simulink model "Visualisation"  (R2023a)
settings: Solver=VariableStepAuto  StartTime=0.0  StopTime=10.0  RelTol=1e-3
values from neighbouring files (symbols this model uses):
  A_long = inv(P_long) * Q_long    [parameters_ctrl.m]
  B_long = inv(P_long) * R_long    [parameters_ctrl.m]
  C_long = eye(4)    [parameters_ctrl.m]
  D_long = zeros(4,2)    [parameters_ctrl.m]
undefined symbols (not defined in the file or in its folder): A_lat, B_lat, C_lat, D_lat
libraries: simulink x2, vrlib x1
settings Model: Creator=simon  LastModifiedBy=simon
settings OptimizationCC: ReuseModelBlockBuffer=off

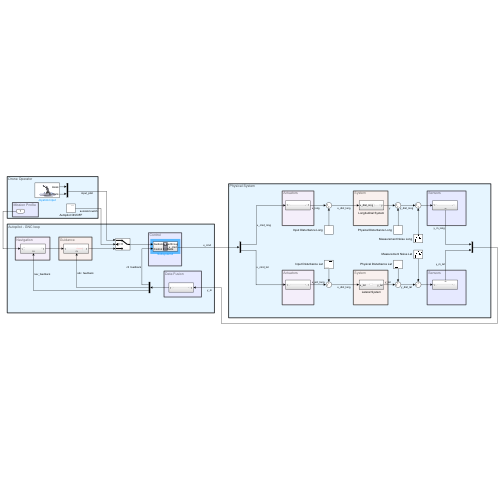
[thumbnail: Simulink's stored preview of the top-level diagram]
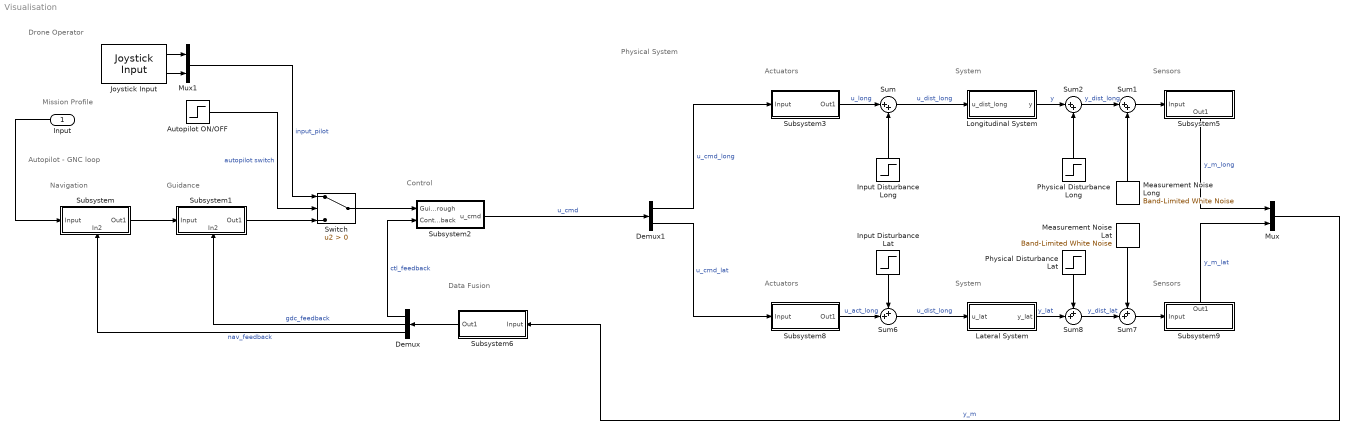
== system Visualisation ==
  note: Drone Operator
  note: Physical System
  note: Autopilot - GNC loop
  note: Navigation
  note: Mission Profile
  note: Guidance
  note: Control
  note: Data Fusion
  note: Actuators
  note: System
  note: Sensors
  note: Sensors
  note: System
  note: Actuators
  Input : Inport
  Autopilot ON/OFF : Step  SampleTime=0
  Demux : Demux  Outputs=3
  Demux1 : Demux  Outputs=2
  Input Disturbance Lat : Step  SampleTime=0
  Input Disturbance Long : Step  SampleTime=0
  Joystick Input : vrlib/Joystick Input  joyid=1  adjustports=on  forcefeed=off
  Lateral System : Subsystem
  Longitudinal System : Subsystem
  Measurement Noise Lat : simulink/Sources/Band-Limited White Noise  Cov=[0.1]  Ts=0.1  seed=[23341]
  Measurement Noise Long : simulink/Sources/Band-Limited White Noise  Cov=[0.1]  Ts=0.1  seed=[23341]
  Mux : Mux  Inputs=2
  Mux1 : Mux  Inputs=2
  Physical Disturbance Lat : Step  SampleTime=0
  Physical Disturbance Long : Step  SampleTime=0
  Subsystem : Subsystem
      settings: PortSchema="{\"entries\":[{\"content\":{\"sides\":[{\"content\":{\"connectorIds\":[\"In1\"]},\"type\":\"ConnectorPlacement.EquallySpacedRectSide\",\"uuid\":\"b55c321e-6281-45a5-aa96-a8b4b9a904a2\"},{\"content\":{\"connectorIds\":[\"Out1\"],\"side\":\"RIGHT\"},\"type\":\"ConnectorPlacement.EquallySpacedRectSide\",\"uuid\":\"1acfb3ee-82d1-4624-97ca-4ff12c3c13a9\"},{\"content\":{\"side\":\"TOP\"},\"type\":\"ConnectorPlacement.EquallySpacedRectSide\",\"uuid\":\"e43a3246-7b87-4c39-ab7c-07bd34ecd1c3\"},{\"content\":{\"connectorIds\":[\"In2\"],\"side\":\"BOTTOM\"},\"type\":\"ConnectorPlacement.EquallySpacedRectSide\",\"uuid\":\"a296ef05-0bf2-440a-9974-10a45cf72fb1\"}]},\"type\":\"ConnectorPlacement.EquallySpacedConnector\",\"uuid\":\"140a1a7e-2a00-4d9b-85bf-b1c0a6988ae3\"}],\"packageUris\":[\"http://schema.mathworks.com/mf0/Connector/R2020b\"],\"version\":\"1.0\"}"
  Subsystem1 : Subsystem
      settings: PortSchema="{\"entries\":[{\"content\":{\"sides\":[{\"content\":{\"connectorIds\":[\"In1\"]},\"type\":\"ConnectorPlacement.EquallySpacedRectSide\",\"uuid\":\"2eb23210-3dea-4b77-a9d4-7110bad0c58c\"},{\"content\":{\"connectorIds\":[\"Out1\"],\"side\":\"RIGHT\"},\"type\":\"ConnectorPlacement.EquallySpacedRectSide\",\"uuid\":\"94c709a1-e7e1-4346-819b-fd02519f91fd\"},{\"content\":{\"connectorIds\":[],\"side\":\"TOP\"},\"type\":\"ConnectorPlacement.EquallySpacedRectSide\",\"uuid\":\"53af2cc2-9550-447d-847d-ecbf9bed457e\"},{\"content\":{\"connectorIds\":[\"In2\"],\"side\":\"BOTTOM\"},\"type\":\"ConnectorPlacement.EquallySpacedRectSide\",\"uuid\":\"c0cb6d07-421f-4c5f-9ed6-902a152412e2\"}]},\"type\":\"ConnectorPlacement.EquallySpacedConnector\",\"uuid\":\"16662f53-7def-47cf-8bdf-f2fc9af7dce9\"}],\"packageUris\":[\"http://schema.mathworks.com/mf0/Connector/R2020b\"],\"version\":\"1.0\"}"
  Subsystem2 : Subsystem
  Subsystem3 : Subsystem
  Subsystem5 : Subsystem
      settings: PortSchema="{\"entries\":[{\"content\":{\"sides\":[{\"content\":{\"connectorIds\":[\"In1\"]},\"type\":\"ConnectorPlacement.EquallySpacedRectSide\",\"uuid\":\"2eb23210-3dea-4b77-a9d4-7110bad0c58c\"},{\"content\":{\"connectorIds\":[],\"side\":\"RIGHT\"},\"type\":\"ConnectorPlacement.EquallySpacedRectSide\",\"uuid\":\"94c709a1-e7e1-4346-819b-fd02519f91fd\"},{\"content\":{\"connectorIds\":[],\"side\":\"TOP\"},\"type\":\"ConnectorPlacement.EquallySpacedRectSide\",\"uuid\":\"53af2cc2-9550-447d-847d-ecbf9bed457e\"},{\"content\":{\"connectorIds\":[\"Out1\"],\"side\":\"BOTTOM\"},\"type\":\"ConnectorPlacement.EquallySpacedRectSide\",\"uuid\":\"b1df5d71-6836-4899-8e9d-10bba38a631d\"}]},\"type\":\"ConnectorPlacement.EquallySpacedConnector\",\"uuid\":\"16662f53-7def-47cf-8bdf-f2fc9af7dce9\"}],\"packageUris\":[\"http://schema.mathworks.com/mf0/Connector/R2020b\"],\"version\":\"1.0\"}"
  Subsystem6 : Subsystem
  Subsystem8 : Subsystem
  Subsystem9 : Subsystem
      settings: PortSchema="{\"entries\":[{\"content\":{\"sides\":[{\"content\":{\"connectorIds\":[\"In1\"]},\"type\":\"ConnectorPlacement.EquallySpacedRectSide\",\"uuid\":\"2eb23210-3dea-4b77-a9d4-7110bad0c58c\"},{\"content\":{\"side\":\"RIGHT\"},\"type\":\"ConnectorPlacement.EquallySpacedRectSide\",\"uuid\":\"94c709a1-e7e1-4346-819b-fd02519f91fd\"},{\"content\":{\"connectorIds\":[\"Out1\"],\"side\":\"TOP\"},\"type\":\"ConnectorPlacement.EquallySpacedRectSide\",\"uuid\":\"53af2cc2-9550-447d-847d-ecbf9bed457e\"},{\"content\":{\"side\":\"BOTTOM\"},\"type\":\"ConnectorPlacement.EquallySpacedRectSide\",\"uuid\":\"b1df5d71-6836-4899-8e9d-10bba38a631d\"}]},\"type\":\"ConnectorPlacement.EquallySpacedConnector\",\"uuid\":\"16662f53-7def-47cf-8bdf-f2fc9af7dce9\"}],\"packageUris\":[\"http://schema.mathworks.com/mf0/Connector/R2020b\"],\"version\":\"1.0\"}"
  Sum : Sum  Inputs=|++
  Sum1 : Sum  Inputs=|++
  Sum2 : Sum  Inputs=|++
  Sum6 : Sum  Inputs=++|
  Sum7 : Sum  Inputs=++|
  Sum8 : Sum  Inputs=++|
  Switch : Switch  Criteria=u2 > Threshold  SaturateOnIntegerOverflow=off  InputSameDT=off
  wires:
  Input/1 -> Subsystem/1(Input)
  Subsystem/1(Out1) -> Subsystem1/1(Input)
  Subsystem1/1(Out1) -> Switch/3
  Subsystem3/1(Out1) -> Sum/1  "u_long"
  Longitudinal System/1(y) -> Sum2/1  "y"
  Subsystem5/1(Out1) -> Mux/1  "y_m_long"
  Subsystem6/1(Out1) -> Demux/1
  Mux1/1 -> Switch/1  "input_pilot"
  Autopilot ON/OFF/1 -> Switch/2  "autopilot switch"
  Input Disturbance Long/1 -> Sum/2
  Sum/1 -> Longitudinal System/1(u_dist_long)  "u_dist_long"
  Measurement Noise Long/1 -> Sum1/2
  Sum1/1 -> Subsystem5/1(Input)
  Physical Disturbance Long/1 -> Sum2/2
  Sum2/1 -> Sum1/1  "y_dist_long"
  Joystick Input/1 -> Mux1/1
  Joystick Input/2 -> Mux1/2
  Demux/2 -> Subsystem1/2(In2)  "gdc_feedback"
  Demux/3 -> Subsystem/2(In2)  "nav_feedback"
  Demux/1 -> Subsystem2/2(Control feedback)  "ctl_feedback"
  Demux1/1 -> Subsystem3/1(Input)  "u_cmd_long"
  Subsystem2/1(u_cmd) -> Demux1/1  "u_cmd"
  Mux/1 -> Subsystem6/1(Input)  "y_m"
  Sum8/1 -> Sum7/2  "y_dist_lat"
  Subsystem9/1(Out1) -> Mux/2  "y_m_lat"
  Physical Disturbance Lat/1 -> Sum8/1
  Sum7/1 -> Subsystem9/1(Input)
  Measurement Noise Lat/1 -> Sum7/1
  Lateral System/1(y_lat) -> Sum8/2  "y_lat"
  Demux1/2 -> Subsystem8/1(Input)  "u_cmd_lat"
  Subsystem8/1(Out1) -> Sum6/2  "u_act_long"
  Input Disturbance Lat/1 -> Sum6/1
  Sum6/1 -> Lateral System/1(u_lat)  "u_dist_long"
  Switch/1 -> Subsystem2/1(Guidance feedthrough)

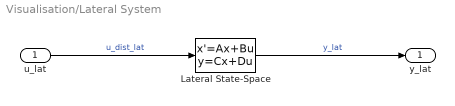
== system Visualisation/Lateral System ==
  u_lat : Inport
  Lateral State-Space : StateSpace  A=A_lat  B=B_lat  C=C_lat  D=D_lat  InitialCondition=0
  y_lat : Outport
  wires:
  u_lat/1 -> Lateral State-Space/1  "u_dist_lat"
  Lateral State-Space/1 -> y_lat/1  "y_lat"

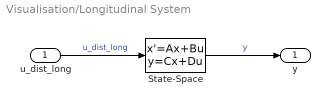
== system Visualisation/Longitudinal System ==
  u_dist_long : Inport
  State-Space : StateSpace  A=A_long  B=B_long  C=C_long  D=D_long  InitialCondition=0
  y : Outport
  wires:
  State-Space/1 -> y/1  "y"
  u_dist_long/1 -> State-Space/1  "u_dist_long"

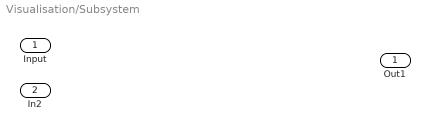
== system Visualisation/Subsystem ==
  Input : Inport
  In2 : Inport  Port=2
  Out1 : Outport

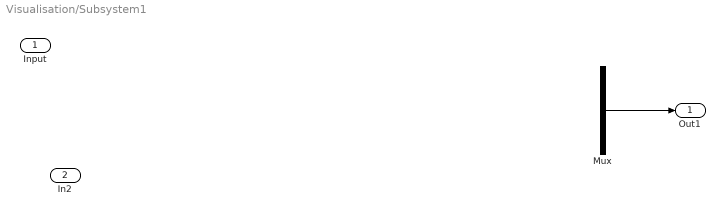
== system Visualisation/Subsystem1 ==
  Input : Inport
  In2 : Inport  Port=2
  Mux : Mux  Inputs=3
  Out1 : Outport
  wires:
  ? -> Mux/1  "h_desired"
  Mux/1 -> Out1/1
  ? -> Mux/2  "v_desired"
  ? -> Mux/3  "chi_desired"

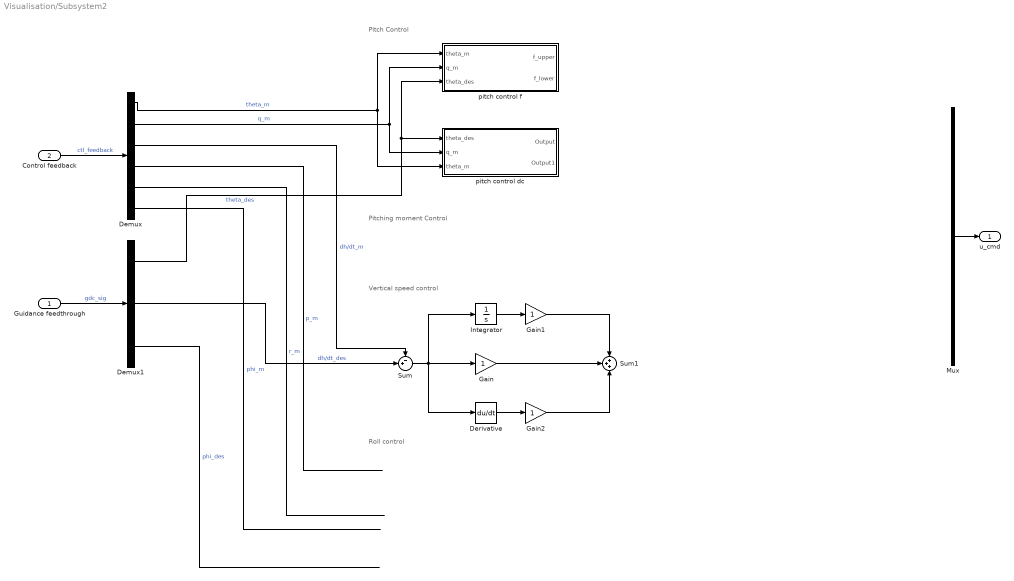
== system Visualisation/Subsystem2 ==
  note: Pitch Control
  note: Pitching moment Control
  note: Vertical speed control
  note: Roll control
  Guidance feedthrough : Inport
  Control feedback : Inport  Port=2
  Demux : Demux  Outputs=6
  Demux1 : Demux  Outputs=3
  Derivative : Derivative
  Gain : Gain
  Gain1 : Gain
  Gain2 : Gain
  Integrator : Integrator
  Mux : Mux  Inputs=12
  Sum : Sum  Inputs=-+|
  Sum1 : Sum  Inputs=+++
  pitch control dc : Subsystem
  pitch control f : Subsystem
  u_cmd : Outport
  wires:
  Control feedback/1 -> Demux/1  "ctl_feedback"
  Demux/3 -> Sum/1  "dh/dt_m"
  Demux/4 -> ?  "p_m"
  Demux/5 -> ?  "r_m"
  Demux/6 -> ?  "phi_m"
  Demux1/3 -> ?  "phi_des"
  Demux1/2 -> Sum/2  "dh/dt_des"
  Guidance feedthrough/1 -> Demux1/1  "gdc_sig"
  Demux/1 -> pitch control f/1(theta_m), pitch control dc/3(theta_m)  "theta_m"
  Demux/2 -> pitch control f/2(q_m), pitch control dc/2(q_m)  "q_m"
  Demux1/1 -> pitch control f/3(theta_des), pitch control dc/1(theta_des)  "theta_des"
  ? -> Mux/1  "f_upper"
  ? -> Mux/2  "f_lower"
  ? -> Mux/3  "dc_upper"
  Mux/1 -> u_cmd/1
  Sum/1 -> Derivative/1, Integrator/1, Gain/1
  Integrator/1 -> Gain1/1
  Derivative/1 -> Gain2/1
  Gain2/1 -> Sum1/3
  Gain/1 -> Sum1/2
  Gain1/1 -> Sum1/1
  ? -> Mux/5  "T"
  ? -> Mux/4  "dc_lower"

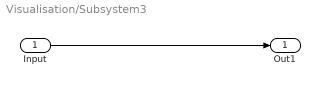
== system Visualisation/Subsystem3 ==
  Input : Inport
  Out1 : Outport
  wires:
  Input/1 -> Out1/1

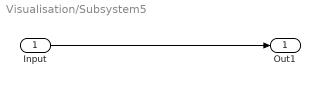
== system Visualisation/Subsystem5 ==
  Input : Inport
  Out1 : Outport
  wires:
  Input/1 -> Out1/1

== system Visualisation/Subsystem6 ==
  Input : Inport
  Out1 : Outport
  wires:
  Input/1 -> Out1/1

== system Visualisation/Subsystem8 ==
  Input : Inport
  Out1 : Outport
  wires:
  Input/1 -> Out1/1

== system Visualisation/Subsystem9 ==
  Input : Inport
  Out1 : Outport
  wires:
  Input/1 -> Out1/1

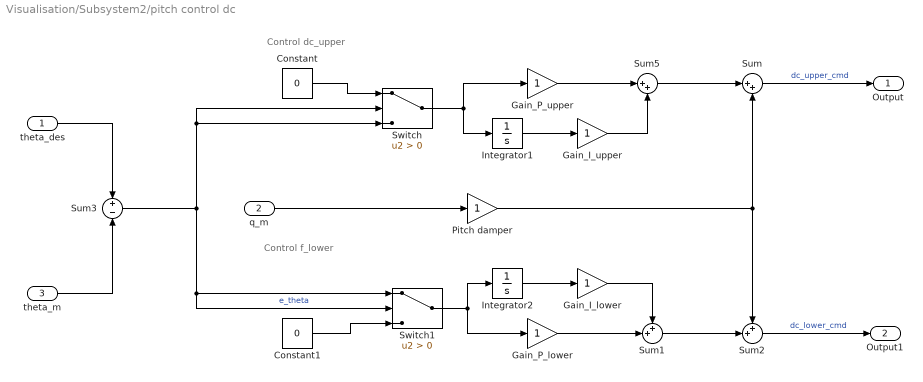
== system Visualisation/Subsystem2/pitch control dc ==
  note: Control f_lower
  note: Control dc_upper
  theta_des : Inport
  q_m : Inport  Port=2
  theta_m : Inport  Port=3
  Constant : Constant  Value=0
  Constant1 : Constant  Value=0
  Gain_I_lower : Gain
  Gain_I_upper : Gain
  Gain_P_lower : Gain
  Gain_P_upper : Gain
  Integrator1 : Integrator
  Integrator2 : Integrator
  Pitch damper : Gain
  Sum : Sum  Inputs=|++
  Sum1 : Sum  Inputs=++|
  Sum2 : Sum  Inputs=++|
  Sum3 : Sum  Inputs=+-
  Sum5 : Sum  Inputs=|++
  Switch : Switch  Criteria=u2 > Threshold  SaturateOnIntegerOverflow=off  InputSameDT=off
  Switch1 : Switch  Criteria=u2 > Threshold  SaturateOnIntegerOverflow=off  InputSameDT=off
  Output : Outport
  Output1 : Outport  Port=2
  wires:
  theta_m/1 -> Sum3/2
  q_m/1 -> Pitch damper/1
  theta_des/1 -> Sum3/1
  Sum3/1 -> Switch1/2, Switch1/1, Switch/2, Switch/3  "e_theta"
  Pitch damper/1 -> Sum2/1, Sum/2
  Sum2/1 -> Output1/1  "dc_lower_cmd"
  Sum/1 -> Output/1  "dc_upper_cmd"
  Sum1/1 -> Sum2/2
  Sum5/1 -> Sum/1
  Gain_I_upper/1 -> Sum5/2
  Gain_P_upper/1 -> Sum5/1
  Integrator1/1 -> Gain_I_upper/1
  Switch/1 -> Gain_P_upper/1, Integrator1/1
  Constant/1 -> Switch/1
  Integrator2/1 -> Gain_I_lower/1
  Gain_I_lower/1 -> Sum1/1
  Gain_P_lower/1 -> Sum1/2
  Constant1/1 -> Switch1/3
  Switch1/1 -> Gain_P_lower/1, Integrator2/1

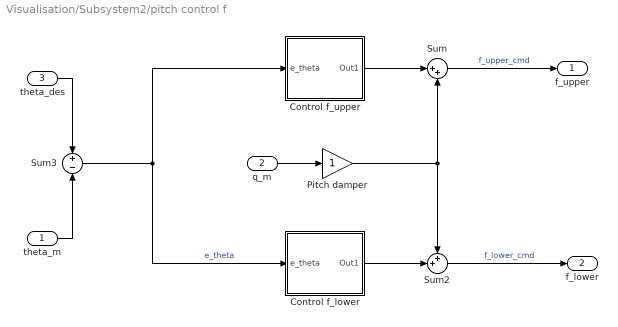
== system Visualisation/Subsystem2/pitch control f ==
  theta_m : Inport
  q_m : Inport  Port=2
  theta_des : Inport  Port=3
  Control f_lower : Subsystem
  Control f_upper : Subsystem
  Pitch damper : Gain
  Sum : Sum  Inputs=|++
  Sum2 : Sum  Inputs=++|
  Sum3 : Sum  Inputs=+-
  f_upper : Outport
  f_lower : Outport  Port=2
  wires:
  theta_m/1 -> Sum3/2
  q_m/1 -> Pitch damper/1
  theta_des/1 -> Sum3/1
  Sum3/1 -> Control f_upper/1(e_theta), Control f_lower/1(e_theta)  "e_theta"
  Pitch damper/1 -> Sum2/1, Sum/2
  Sum2/1 -> f_lower/1  "f_lower_cmd"
  Sum/1 -> f_upper/1  "f_upper_cmd"
  Control f_lower/1(Out1) -> Sum2/2
  Control f_upper/1(Out1) -> Sum/1

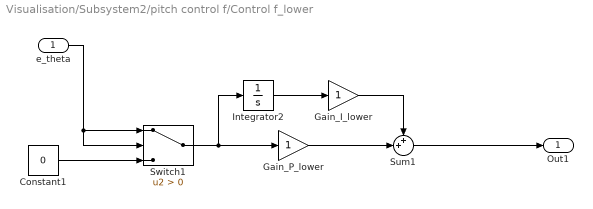
== system Visualisation/Subsystem2/pitch control f/Control f_lower ==
  e_theta : Inport
  Constant1 : Constant  Value=0
  Gain_I_lower : Gain
  Gain_P_lower : Gain
  Integrator2 : Integrator
  Sum1 : Sum  Inputs=++|
  Switch1 : Switch  Criteria=u2 > Threshold  SaturateOnIntegerOverflow=off  InputSameDT=off
  Out1 : Outport
  wires:
  Switch1/1 -> Integrator2/1, Gain_P_lower/1
  Constant1/1 -> Switch1/3
  e_theta/1 -> Switch1/1, Switch1/2
  Sum1/1 -> Out1/1
  Gain_P_lower/1 -> Sum1/2
  Gain_I_lower/1 -> Sum1/1
  Integrator2/1 -> Gain_I_lower/1

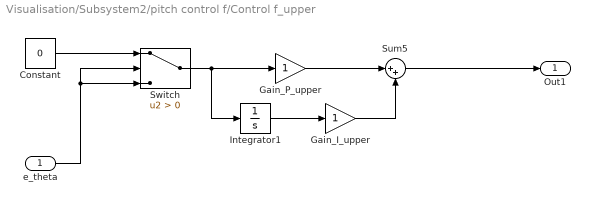
== system Visualisation/Subsystem2/pitch control f/Control f_upper ==
  e_theta : Inport
  Constant : Constant  Value=0
  Gain_I_upper : Gain
  Gain_P_upper : Gain
  Integrator1 : Integrator
  Sum5 : Sum  Inputs=|++
  Switch : Switch  Criteria=u2 > Threshold  SaturateOnIntegerOverflow=off  InputSameDT=off
  Out1 : Outport
  wires:
  Constant/1 -> Switch/1
  Switch/1 -> Integrator1/1, Gain_P_upper/1
  Sum5/1 -> Out1/1
  Integrator1/1 -> Gain_I_upper/1
  Gain_P_upper/1 -> Sum5/1
  e_theta/1 -> Switch/2, Switch/3
  Gain_I_upper/1 -> Sum5/2
